simulink model "Force_Position"  (R2015b)
settings: Solver=FixedStepAuto  StartTime=0.0  StopTime=10  FixedStep=Ts  RelTol=1e-3
values from neighbouring files (symbols this model uses):
  b = block.DialogPrm(1).Data    [controller_less.m]    (also in controller_more.m)
  S = [S;Km, Ks, Pm, Ps, Bm, Bs]    [Gains.m]
undefined symbols (not defined in the file or in its folder): Dm, Ds, Gamma, Kdp, Kpp, Ts
settings Model: Creator=TOSHIBA  LastModifiedBy=TOSHIBA

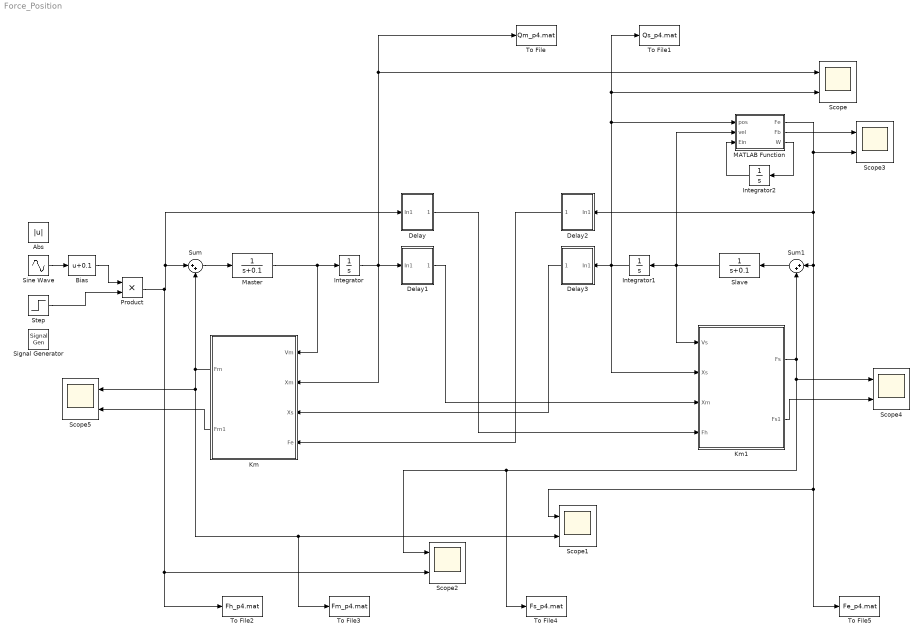
== system Force_Position ==
  Abs : Abs
  Bias : Bias  Bias=0.1
  Delay : Subsystem
  Delay1 : Subsystem
  Delay2 : Subsystem
  Delay3 : Subsystem
  Integrator : Integrator
  Integrator1 : Integrator
  Integrator2 : Integrator
  Km : Subsystem
  Km1 : Subsystem
  MATLAB Function : MATLAB Function  TreatAsAtomicUnit=on
  Master : TransferFcn  Denominator=[1 0.1]
  Product : Product
  Scope{,1..5} (6 alike) : Scope  NumInputPorts=2
  Signal Generator : SignalGenerator  WaveForm=square  Amplitude=-1  Frequency=0.05*pi  Units=rad/sec
  Sine Wave : Sin  Amplitude=2  Frequency=pi/2  SampleTime=0
  Slave : TransferFcn  Denominator=[1 0.1]
  Step : Step  Time=20  Before=1  After=0  SampleTime=0
  Sum : Sum  Inputs=|++
  Sum1 : Sum  Inputs=|++
  To File : ToFile  Filename=Qm_p4.mat  MatrixName=Qm_p4  SaveFormat=Timeseries
  To File1 : ToFile  Filename=Qs_p4.mat  MatrixName=Qs_p4  SaveFormat=Timeseries
  To File2 : ToFile  Filename=Fh_p4.mat  MatrixName=Fh_p4  SaveFormat=Timeseries
  To File3 : ToFile  Filename=Fm_p4.mat  MatrixName=Fm_p4  SaveFormat=Timeseries
  To File4 : ToFile  Filename=Fs_p4.mat  MatrixName=Fs_p4  SaveFormat=Timeseries
  To File5 : ToFile  Filename=Fe_p4.mat  MatrixName=Fe_p4  SaveFormat=Timeseries
  wires:
  Sum/1 -> Master/1
  Master/1 -> Km/1(Vm), Integrator/1
  Integrator/1 -> Delay1/1(In1), Km/2(Xm), To File/1, Scope/1
  Km/1(Fm) -> Scope5/1, To File3/1, Scope1/2, Sum/2
  Slave/1 -> MATLAB Function/2(vel), Km1/1(Vs), Integrator1/1
  Km1/1(Fs) -> Scope4/1, To File4/1, Scope2/1, Sum1/2
  Sum1/1 -> Slave/1
  Delay1/1(Out1) -> Km1/3(Xm)
  Delay3/1(Out1) -> Km/3(Xs)
  Delay2/1(Out1) -> Km/4(Fe)
  Delay/1(Out1) -> Km1/4(Fh)
  Integrator1/1 -> Delay3/1(In1), MATLAB Function/1(pos), To File1/1, Scope/2, Km1/2(Xs)
  MATLAB Function/1(Fe) -> Delay2/1(In1), To File5/1, Scope1/1, Sum1/1, Scope3/2
  MATLAB Function/3(W) -> Integrator2/1
  Integrator2/1 -> MATLAB Function/3(Ein)
  MATLAB Function/2(Fb) -> Scope3/1
  Sine Wave/1 -> Bias/1
  Bias/1 -> Product/1
  Product/1 -> To File2/1, Scope2/2, Delay/1(In1), Sum/1
  Step/1 -> Product/2
  Km1/2(Fs1) -> Scope4/2
  Km/2(Fm1) -> Scope5/2

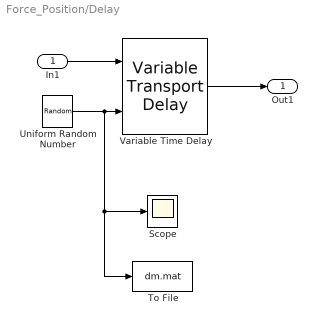
== system Force_Position/Delay ==
  In1 : Inport
  Scope : Scope
  To File : ToFile  Filename=dm.mat  MatrixName=dm  SaveFormat=Timeseries
  Uniform Random Number : UniformRandomNumber  Minimum=0  Maximum=Dm  SampleTime=Ts
  Variable Time Delay : VariableTransportDelay  MaximumDelay=Dm
  Out1 : Outport
  wires:
  Uniform Random Number/1 -> To File/1, Scope/1, Variable Time Delay/2
  In1/1 -> Variable Time Delay/1
  Variable Time Delay/1 -> Out1/1

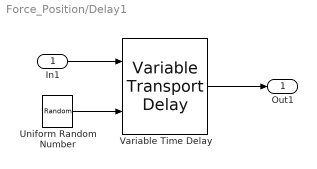
== system Force_Position/Delay1 ==
  In1 : Inport
  Uniform Random Number : UniformRandomNumber  Minimum=0  Maximum=Dm  SampleTime=Ts
  Variable Time Delay : VariableTransportDelay  MaximumDelay=Dm
  Out1 : Outport
  wires:
  Variable Time Delay/1 -> Out1/1
  In1/1 -> Variable Time Delay/1
  Uniform Random Number/1 -> Variable Time Delay/2

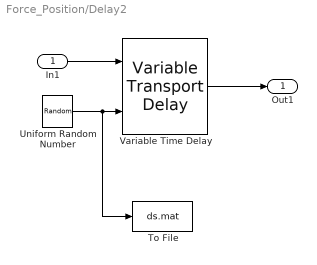
== system Force_Position/Delay2 ==
  In1 : Inport
  To File : ToFile  Filename=ds.mat  MatrixName=ds  SaveFormat=Timeseries
  Uniform Random Number : UniformRandomNumber  Minimum=0  Maximum=Ds  SampleTime=Ts
  Variable Time Delay : VariableTransportDelay  MaximumDelay=Ds
  Out1 : Outport
  wires:
  Variable Time Delay/1 -> Out1/1
  In1/1 -> Variable Time Delay/1
  Uniform Random Number/1 -> To File/1, Variable Time Delay/2

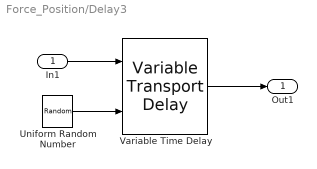
== system Force_Position/Delay3 ==
  In1 : Inport
  Uniform Random Number : UniformRandomNumber  Minimum=0  Maximum=Ds  SampleTime=Ts
  Variable Time Delay : VariableTransportDelay  MaximumDelay=Ds
  Out1 : Outport
  wires:
  Uniform Random Number/1 -> Variable Time Delay/2
  In1/1 -> Variable Time Delay/1
  Variable Time Delay/1 -> Out1/1

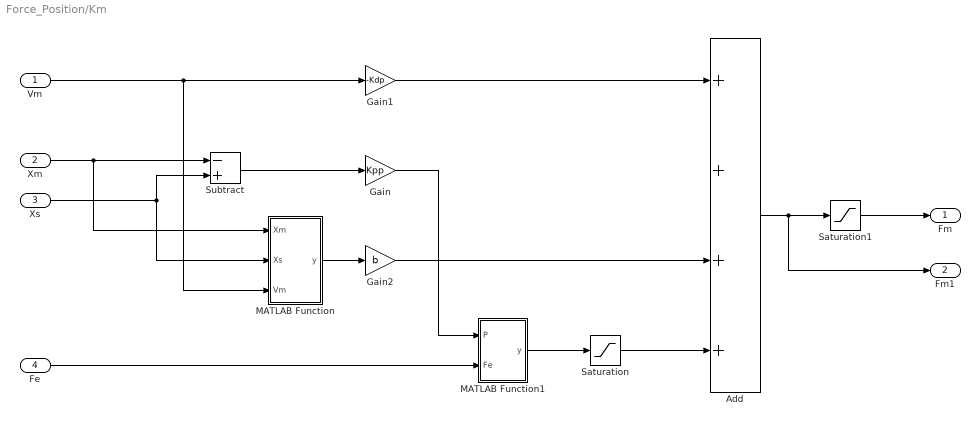
== system Force_Position/Km ==
  Vm : Inport
  Xm : Inport  Port=2
  Xs : Inport  Port=3
  Fe : Inport  Port=4
  Add : Sum  Inputs=++++
  Gain : Gain  Gain=Kpp
  Gain1 : Gain  Gain=-Kdp
  Gain2 : Gain  Gain=b
  MATLAB Function : MATLAB Function  TreatAsAtomicUnit=on
  MATLAB Function1 : MATLAB Function  TreatAsAtomicUnit=on
  Saturation : Saturate  UpperLimit=Gamma  LowerLimit=-Gamma  ZeroCross=off
  Saturation1 : Saturate  UpperLimit=S  LowerLimit=-S  ZeroCross=off
  Subtract : Sum  Inputs=-+
  Fm : Outport
  Fm1 : Outport  Port=2
  wires:
  Xm/1 -> MATLAB Function/1(Xm), Subtract/1
  Xs/1 -> Subtract/2, MATLAB Function/2(Xs)
  Gain1/1 -> Add/1
  Add/1 -> Fm1/1, Saturation1/1
  Vm/1 -> MATLAB Function/3(Vm), Gain1/1
  Subtract/1 -> Gain/1
  MATLAB Function/1(y) -> Gain2/1
  Gain2/1 -> Add/3
  Saturation1/1 -> Fm/1
  MATLAB Function1/1(y) -> Saturation/1
  Fe/1 -> MATLAB Function1/2(Fe)
  Gain/1 -> MATLAB Function1/1(P)
  Saturation/1 -> Add/4

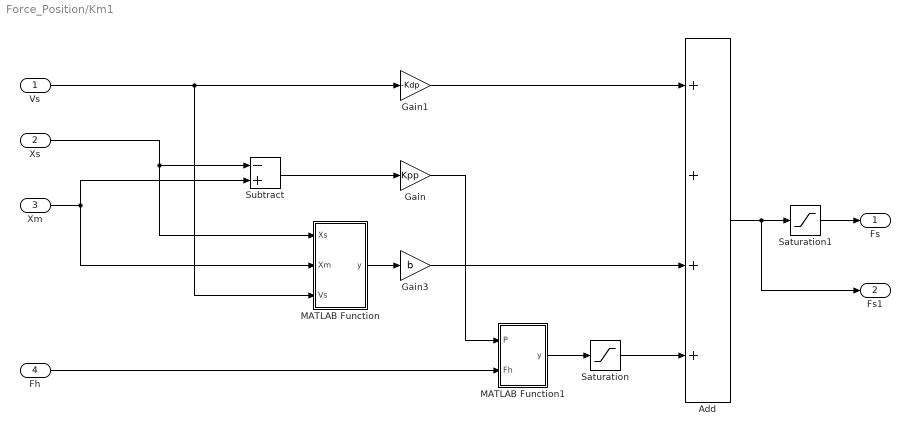
== system Force_Position/Km1 ==
  Vs : Inport
  Xs : Inport  Port=2
  Xm : Inport  Port=3
  Fh : Inport  Port=4
  Add : Sum  Inputs=++++
  Gain : Gain  Gain=Kpp
  Gain1 : Gain  Gain=-Kdp
  Gain3 : Gain  Gain=b
  MATLAB Function : MATLAB Function  TreatAsAtomicUnit=on
  MATLAB Function1 : MATLAB Function  TreatAsAtomicUnit=on
  Saturation : Saturate  UpperLimit=Gamma  LowerLimit=-Gamma  ZeroCross=off
  Saturation1 : Saturate  UpperLimit=S  LowerLimit=-S  ZeroCross=off
  Subtract : Sum  Inputs=-+
  Fs : Outport
  Fs1 : Outport  Port=2
  wires:
  Xs/1 -> MATLAB Function/1(Xs), Subtract/1
  Xm/1 -> Subtract/2, MATLAB Function/2(Xm)
  Subtract/1 -> Gain/1
  Vs/1 -> MATLAB Function/3(Vs), Gain1/1
  Gain1/1 -> Add/1
  Add/1 -> Fs1/1, Saturation1/1
  MATLAB Function/1(y) -> Gain3/1
  Gain3/1 -> Add/3
  Saturation1/1 -> Fs/1
  MATLAB Function1/1(y) -> Saturation/1
  Fh/1 -> MATLAB Function1/2(Fh)
  Gain/1 -> MATLAB Function1/1(P)
  Saturation/1 -> Add/4

== matlab function Force_Position/Km/MATLAB Function ==
  data: Xm input; y output; Xs input; Vm input
function y = fcn(Xm,Xs,Vm)
%#codegen
if Vm>0.01
    y=((Xm-Xs)^2)/Vm;
else
    y=0;
end

== matlab function Force_Position/MATLAB Function ==
  data: pos input; vel input; Fe output; Fb output; Ein input; W output
function [Fe, Fb, W] = Envir(pos,vel,Ein)
%#codegen
kWall = 10000;
bWall = 0;
if pos>=0.1
    Fk=-(pos-0.1)*kWall;
    if Ein<=1
        Fb=bWall*vel;
    else
        Fb=0;
    end
    Fe=Fk+Fb;
    W=Fb*vel;
else
    Fe=0;
    Fb=0;
    W=0;
end

== matlab function Force_Position/Km1/MATLAB Function ==
  data: Xs input; Xm input; y output; Vs input
function y = fcn(Xs,Xm,Vs)
%#codegen
if Vs>0.01
    y=((Xs-Xm)^2)/Vs;
else
    y=0;
end

== matlab function Force_Position/Km/MATLAB Function1 ==
  data: P input; y output; Fe input
function y = fcn(P,Fe)
%#codegen
if abs(Fe)<=abs(P)
    y=P+Fe;
else
    if Fe*P>=0
        y=2*P;
    else
        y=0;
    end
end

== matlab function Force_Position/Km1/MATLAB Function1 ==
  data: P input; y output; Fh input
function y = fcn(P,Fh)
%#codegen
if abs(Fh)<=abs(P)
    y=P+Fh;
else
    if P*Fh>0
        y=2*P;
    else
        y=0;
    end
end
